simulink model "nn_fuel_control_3_15"  (R2021a)
settings: Solver=ode15s  StartTime=0.0  StopTime=T  MaxStep=.01  RelTol=1e-3
undefined symbols (not defined in the file): AF_sensor_tol, fault_time, fuel_inj_tol, kappa_tol, MAF_sensor_tol, pump_tol, tau_ww_tol
libraries: neural x50
(part 2 of 2)

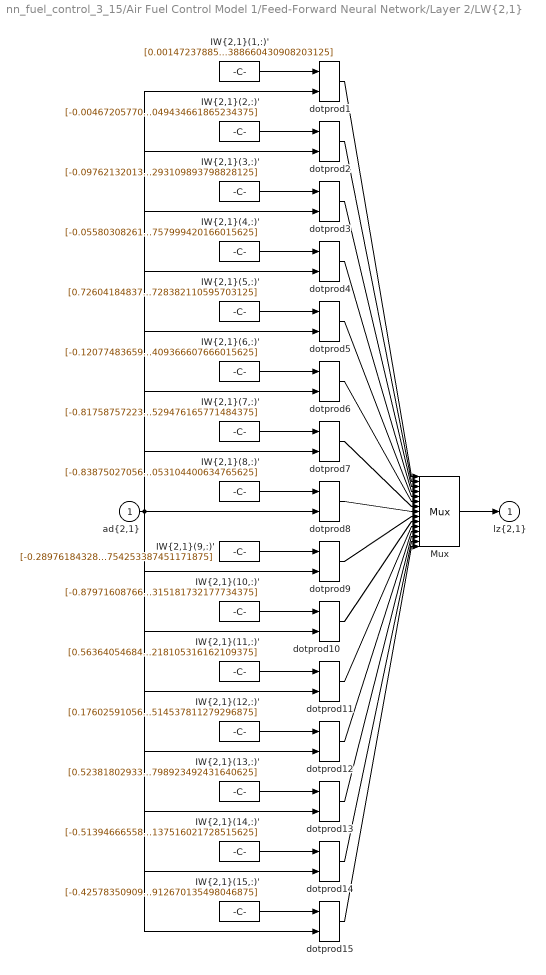
== system nn_fuel_control_3_15/Air Fuel Control Model 1/Feed-Forward Neural Network/Layer 2/LW{2,1} ==
  "ad{2,1}" : Inport  PortDimensions=15
      mask Display: e = 0.06;c1 = [120 230 180]/255;c2 = ([120 230 180]+0)/(256+128);c3 = ([120 230 180]+128)/(256+128);patch([0 1 1 0],[0 0 1 1],c1);patch([0 1 1 1-e 1-e 0+e],[0 0 1 1-e 0+e 0+e],c2);patch([0 0 1 1-e 0+e 0+e],[0 1 1 1-e 1-e 0+e],c3);plot([0 1 1 0 0],[0 0 1 1 0]);
  "IW{2,1}(1,:)'" : Constant  Value=[0.0014723788564683371049568449961952865123748779296875;-0.4105035744953438037185833309195004403591156005859375;0.92504607137404970540472959328326396644115447998046875;-0.13140968467763602944842205033637583255767822265625;0.88617470350879212759309666580520570278167724609375;0.10943690712673904974483463092838064767420291900634765625;0.8357847560107405371354616363532841205596923828125;-0.1424217355145691865647705753872287459671497344970703125;-0.9683741182261533797515085097984410822391510009765625;0.2078972828309095521870375478101777844130992889404296875;-0.141657891245238809485584852154715918004512786865234375;0.2854467052004372451534663923666812479496002197265625;-0.47802444452566505983526212730794213712215423583984375;0.007742822605644341001085440012730032321996986865997314453125;0.7026691591665628067175930482335388660430908203125]
      mask Display: e = 0.06;c1 = [120 150 230]/255;c2 = ([120 150 230]+0)/383;c3 = ([120 150 230]+128)/383;patch([0 1 1 0],[0 0 1 1],c1);patch([0 1 1 1-e 1-e 0+e],[0 0 1 1-e 0+e 0+e],c2);patch([0 0 1 1-e 0+e 0+e],[0 1 1 1-e 1-e 0+e],c3);plot([0 1 1 0 0],[0 0 1 1 0]);disp('weights');
  "IW{2,1}(10,:)'" : Constant  Value=[-0.8797160876685172770095277883228845894336700439453125;0.789339370544755780656487331725656986236572265625;-0.7233137151600008696306076672044582664966583251953125;0.6015191081513704407512932448298670351505279541015625;-0.11263426835994684582775704484447487629950046539306640625;0.8415776576411524434462307908688671886920928955078125;-0.2980449987010034273993142051040194928646087646484375;-0.171843305813586422203798065311275422573089599609375;0.117265923905212565703237714842543937265872955322265625;0.30307170949009909488580660763545893132686614990234375;-0.293941626387824062049958229181356728076934814453125;-0.03082063515976596335121939773671329021453857421875;-0.9050983525641178584209001201088540256023406982421875;-0.99163442468549334307681419886648654937744140625;0.521943270434400030666211023344658315181732177734375]
      mask Display: e = 0.06;c1 = [120 150 230]/255;c2 = ([120 150 230]+0)/383;c3 = ([120 150 230]+128)/383;patch([0 1 1 0],[0 0 1 1],c1);patch([0 1 1 1-e 1-e 0+e],[0 0 1 1-e 0+e 0+e],c2);patch([0 0 1 1-e 0+e 0+e],[0 1 1 1-e 1-e 0+e],c3);plot([0 1 1 0 0],[0 0 1 1 0]);disp('weights');
  "IW{2,1}(11,:)'" : Constant  Value=[0.5636405468410743413443242388893850147724151611328125;-0.6000555782086010037090773039381019771099090576171875;-0.9083589997321432907284588509355671703815460205078125;-0.039439145748280335368463056511245667934417724609375;-0.360599567968600986933580543336574919521808624267578125;-0.9013962864403468611129710552631877362728118896484375;0.818131379099671374177660254645161330699920654296875;0.2148021088713241433243439360012416727840900421142578125;-0.6090730591420296935467604271252639591693878173828125;-0.490614841968887549494837685415404848754405975341796875;0.87058254048700034477548115319223143160343170166015625;0.9743140261337905894123423422570340335369110107421875;-0.231388861045130678206760421744547784328460693359375;-0.81143184376103416610703789046965539455413818359375;0.7149273616405726894384997649467550218105316162109375]
      mask Display: e = 0.06;c1 = [120 150 230]/255;c2 = ([120 150 230]+0)/383;c3 = ([120 150 230]+128)/383;patch([0 1 1 0],[0 0 1 1],c1);patch([0 1 1 1-e 1-e 0+e],[0 0 1 1-e 0+e 0+e],c2);patch([0 0 1 1-e 0+e 0+e],[0 1 1 1-e 1-e 0+e],c3);plot([0 1 1 0 0],[0 0 1 1 0]);disp('weights');
  "IW{2,1}(12,:)'" : Constant  Value=[0.176025910561064424797450556070543825626373291015625;0.8938959851841807857653066093917004764080047607421875;0.23024565712716604792831276427023112773895263671875;0.5912002453814280134025693769217468798160552978515625;-0.13767899499483693404044970520772039890289306640625;0.39561104597748197875262121669948101043701171875;-0.551936271474654294166839463287033140659332275390625;-0.3033516443932107176095769318635575473308563232421875;-0.7286060567887997496683283316087909042835235595703125;-0.7412289835134810989103471001726575195789337158203125;0.40006283904586847910422875429503619670867919921875;-0.4572149619781218365943686876562424004077911376953125;-0.92336675575178883690341535839252173900604248046875;0.4141772355500019653362642202409915626049041748046875;-0.697359994923690162949014847981743514537811279296875]
      mask Display: e = 0.06;c1 = [120 150 230]/255;c2 = ([120 150 230]+0)/383;c3 = ([120 150 230]+128)/383;patch([0 1 1 0],[0 0 1 1],c1);patch([0 1 1 1-e 1-e 0+e],[0 0 1 1-e 0+e 0+e],c2);patch([0 0 1 1-e 0+e 0+e],[0 1 1 1-e 1-e 0+e],c3);plot([0 1 1 0 0],[0 0 1 1 0]);disp('weights');
  "IW{2,1}(13,:)'" : Constant  Value=[0.5238180293357050931746243804809637367725372314453125;0.4144582229988842403400894909282214939594268798828125;-0.71210330551954204025832950719632208347320556640625;-0.2764686429265024170121023416868411004543304443359375;0.84370835682129097232717640508781187236309051513671875;-0.58371761794929810651666457488317973911762237548828125;-0.647040471028641928086244661244563758373260498046875;-0.0257292770502409000321630827556873555295169353485107421875;-0.109912687998933000788071012721047736704349517822265625;0.41116241447809154241355145131819881498813629150390625;-0.55283670379326566024502653817762620747089385986328125;0.7529229726831230262718008816591463983058929443359375;0.15049080269142611765431638559675775468349456787109375;-0.231897338961606302998319506514235399663448333740234375;-0.070382914756523806687482647248543798923492431640625]
      mask Display: e = 0.06;c1 = [120 150 230]/255;c2 = ([120 150 230]+0)/383;c3 = ([120 150 230]+128)/383;patch([0 1 1 0],[0 0 1 1],c1);patch([0 1 1 1-e 1-e 0+e],[0 0 1 1-e 0+e 0+e],c2);patch([0 0 1 1-e 0+e 0+e],[0 1 1 1-e 1-e 0+e],c3);plot([0 1 1 0 0],[0 0 1 1 0]);disp('weights');
  "IW{2,1}(14,:)'" : Constant  Value=[-0.5139466655833884178861126201809383928775787353515625;-0.6994970916207192690450256122858263552188873291015625;0.02461016033035413885787789922687807120382785797119140625;-0.2071609556260745055311645046458579599857330322265625;0.62690154518222629409507362652220763266086578369140625;-0.68570881908632952406179583704215474426746368408203125;0.6935255351681650637374332291074097156524658203125;0.2274889095578533637631579722437891177833080291748046875;-0.1208011883769616046091499583781114779412746429443359375;0.61407664799677508238318068833905272185802459716796875;-0.860561180678970583102227465133182704448699951171875;-0.901805715626496695591640673228539526462554931640625;-0.756946189561250815103221611934714019298553466796875;0.2377717869806747208460961928722099401056766510009765625;-0.9584754628916682950290351072908379137516021728515625]
      mask Display: e = 0.06;c1 = [120 150 230]/255;c2 = ([120 150 230]+0)/383;c3 = ([120 150 230]+128)/383;patch([0 1 1 0],[0 0 1 1],c1);patch([0 1 1 1-e 1-e 0+e],[0 0 1 1-e 0+e 0+e],c2);patch([0 0 1 1-e 0+e 0+e],[0 1 1 1-e 1-e 0+e],c3);plot([0 1 1 0 0],[0 0 1 1 0]);disp('weights');
  "IW{2,1}(15,:)'" : Constant  Value=[-0.4257835090962220903065826860256493091583251953125;0.7545482545397168561152057009167037904262542724609375;0.693650957176581872687393115484155714511871337890625;-0.6058271909569750146573596794041804969310760498046875;-0.92243298192882450248220038702129386365413665771484375;0.463413219568864220843096290991525165736675262451171875;0.338649245461934089718170071137137711048126220703125;0.484763807823216097414587011371622793376445770263671875;0.39292867758759653096234387703589163720607757568359375;0.805180629601002895157080274657346308231353759765625;0.2171358898594655528757613183188368566334247589111328125;-0.84680999387249666909838197170756757259368896484375;-0.3689431272830090424719173824996687471866607666015625;-0.62736288244411664294375441386364400386810302734375;-0.1978189326577559636888281602296046912670135498046875]
      mask Display: e = 0.06;c1 = [120 150 230]/255;c2 = ([120 150 230]+0)/383;c3 = ([120 150 230]+128)/383;patch([0 1 1 0],[0 0 1 1],c1);patch([0 1 1 1-e 1-e 0+e],[0 0 1 1-e 0+e 0+e],c2);patch([0 0 1 1-e 0+e 0+e],[0 1 1 1-e 1-e 0+e],c3);plot([0 1 1 0 0],[0 0 1 1 0]);disp('weights');
  "IW{2,1}(2,:)'" : Constant  Value=[-0.004672057704449006365621244185604155063629150390625;0.9755623302918092765168012192589230835437774658203125;-0.2802782291596883634809955765376798808574676513671875;0.530568769281649199598405175493098795413970947265625;-0.3711149592822611253950526588596403598785400390625;-0.6701597425193110968422161022317595779895782470703125;0.48671231916720270049836472026072442531585693359375;-0.7434126313786528772453721103374846279621124267578125;-0.153098699941905724841717528761364519596099853515625;0.85133638949894674397000926546752452850341796875;0.9338773130103581454619643409387208521366119384765625;0.8820582695436858244875111267901957035064697265625;-0.9020048816383496870230374042876064777374267578125;-0.32054209486867168976687025860883295536041259765625;-0.5428806493898130636210908050998114049434661865234375]
      mask Display: e = 0.06;c1 = [120 150 230]/255;c2 = ([120 150 230]+0)/383;c3 = ([120 150 230]+128)/383;patch([0 1 1 0],[0 0 1 1],c1);patch([0 1 1 1-e 1-e 0+e],[0 0 1 1-e 0+e 0+e],c2);patch([0 0 1 1-e 0+e 0+e],[0 1 1 1-e 1-e 0+e],c3);plot([0 1 1 0 0],[0 0 1 1 0]);disp('weights');
  "IW{2,1}(3,:)'" : Constant  Value=[-0.097621320133909339489264311851002275943756103515625;0.2612783169119214932152317487634718418121337890625;-0.055215070832447997462022470926967798732221126556396484375;0.8160125298612683764076791703701019287109375;0.65646477091284527460857134428806602954864501953125;-0.19085913401025933477939133808831684291362762451171875;0.3087414420961487326877659143065102398395538330078125;0.9224876971971227579416563457925803959369659423828125;-0.266571874563814203984435380334616638720035552978515625;0.6702336279486582615305678700678981840610504150390625;0.197265872962691324321582442280487157404422760009765625;-0.57729764225107604858067134045995771884918212890625;-0.791492072672669966237890548654831945896148681640625;0.81667830492291937360960218938998878002166748046875;-0.8911950061504072539975140898604877293109893798828125]
      mask Display: e = 0.06;c1 = [120 150 230]/255;c2 = ([120 150 230]+0)/383;c3 = ([120 150 230]+128)/383;patch([0 1 1 0],[0 0 1 1],c1);patch([0 1 1 1-e 1-e 0+e],[0 0 1 1-e 0+e 0+e],c2);patch([0 0 1 1-e 0+e 0+e],[0 1 1 1-e 1-e 0+e],c3);plot([0 1 1 0 0],[0 0 1 1 0]);disp('weights');
  "IW{2,1}(4,:)'" : Constant  Value=[-0.0558030826137325686175927330623380839824676513671875;0.4347023464860020336431034593260847032070159912109375;0.275440674566879317719525488428189419209957122802734375;-0.25350814443316949109430424869060516357421875;0.381186478547256124560504986220621503889560699462890625;-0.53969236281862009718679473735392093658447265625;0.3138820723565487469386425800621509552001953125;0.314206063773635080327295554525335319340229034423828125;-0.91256989931503273982826840438065119087696075439453125;-0.75671300750665537737660315542598254978656768798828125;-0.1656127582319334712313008139972225762903690338134765625;0.4185309459959771771764280856586992740631103515625;-0.76890276522204448195196846427279524505138397216796875;0.661584923547618330985642387531697750091552734375;-0.3590957813671791232223995393724180757999420166015625]
      mask Display: e = 0.06;c1 = [120 150 230]/255;c2 = ([120 150 230]+0)/383;c3 = ([120 150 230]+128)/383;patch([0 1 1 0],[0 0 1 1],c1);patch([0 1 1 1-e 1-e 0+e],[0 0 1 1-e 0+e 0+e],c2);patch([0 0 1 1-e 0+e 0+e],[0 1 1 1-e 1-e 0+e],c3);plot([0 1 1 0 0],[0 0 1 1 0]);disp('weights');
  "IW{2,1}(5,:)'" : Constant  Value=[0.7260418483791071242450243516941554844379425048828125;-0.2323204701209327094346690500969998538494110107421875;0.58094310317328190507168983458541333675384521484375;-0.10149087657121658168080102768726646900177001953125;0.017385472622406965281793844724234077148139476776123046875;-0.2465918696556105016437498989034793339669704437255859375;-0.065147713611995783367092371918261051177978515625;0.82285250893895656165710761342779733240604400634765625;-0.5632819611943988835633945200243033468723297119140625;-0.79200473782083558038635828779661096632480621337890625;-0.58294595380808889029111696800100617110729217529296875;0.8069688237247607531799076241441071033477783203125;-0.5731754303914218251492229683208279311656951904296875;0.74394758108042580158070222751121036708354949951171875;0.757136590987837809763050245237536728382110595703125]
      mask Display: e = 0.06;c1 = [120 150 230]/255;c2 = ([120 150 230]+0)/383;c3 = ([120 150 230]+128)/383;patch([0 1 1 0],[0 0 1 1],c1);patch([0 1 1 1-e 1-e 0+e],[0 0 1 1-e 0+e 0+e],c2);patch([0 0 1 1-e 0+e 0+e],[0 1 1 1-e 1-e 0+e],c3);plot([0 1 1 0 0],[0 0 1 1 0]);disp('weights');
  "IW{2,1}(6,:)'" : Constant  Value=[-0.1207748365903345000305080247926525771617889404296875;-0.4566001292990182758302353249746374785900115966796875;0.7674321577875711231087052510702051222324371337890625;0.532782020818384882687723802519030869007110595703125;-0.5503302152362241628225092426873743534088134765625;-0.870981104051296473045340462704189121723175048828125;-0.3023547547324063611284827857161872088909149169921875;0.2357299472378218130330651547410525381565093994140625;0.71943294959485815098787497845478355884552001953125;0.892178685051398634442421098356135189533233642578125;-0.264484462101378436926779613713733851909637451171875;0.6035938989327063186607347233803011476993560791015625;0.0123594330541221264496698495349846780300140380859375;-0.00799278345603138262731590657494962215423583984375;-0.71855220021363752636034405441023409366607666015625]
      mask Display: e = 0.06;c1 = [120 150 230]/255;c2 = ([120 150 230]+0)/383;c3 = ([120 150 230]+128)/383;patch([0 1 1 0],[0 0 1 1],c1);patch([0 1 1 1-e 1-e 0+e],[0 0 1 1-e 0+e 0+e],c2);patch([0 0 1 1-e 0+e 0+e],[0 1 1 1-e 1-e 0+e],c3);plot([0 1 1 0 0],[0 0 1 1 0]);disp('weights');
  "IW{2,1}(7,:)'" : Constant  Value=[-0.8175875722366179321198842444573529064655303955078125;-0.905813293112641471083179567358456552028656005859375;-0.3844932577919755178896821234957315027713775634765625;0.2056336354930061727230850010528229176998138427734375;-0.76141972218104125857962571899406611919403076171875;-0.9439776643957298318809989723376929759979248046875;0.6997489290599505640244615278788842260837554931640625;0.8655339347746793254856356725213117897510528564453125;0.4664203946738567641006056874175556004047393798828125;0.0626214973472627445261196044157259166240692138671875;0.4649690508771568975276977653265930712223052978515625;-0.38200351988705794070710908272303640842437744140625;-0.666044497810676983107214255142025649547576904296875;0.9083497414519896562268286288599483668804168701171875;-0.0908783258153691431147080947994254529476165771484375]
      mask Display: e = 0.06;c1 = [120 150 230]/255;c2 = ([120 150 230]+0)/383;c3 = ([120 150 230]+128)/383;patch([0 1 1 0],[0 0 1 1],c1);patch([0 1 1 1-e 1-e 0+e],[0 0 1 1-e 0+e 0+e],c2);patch([0 0 1 1-e 0+e 0+e],[0 1 1 1-e 1-e 0+e],c3);plot([0 1 1 0 0],[0 0 1 1 0]);disp('weights');
  "IW{2,1}(8,:)'" : Constant  Value=[-0.8387502705666316504817814347916282713413238525390625;-0.9869927371518103509373531778692267835140228271484375;-0.049215002141873132046612226986326277256011962890625;-0.6725714957969464169451612178818322718143463134765625;-0.41634711954292225044582664850167930126190185546875;-0.0546792633337906952561979778693057596683502197265625;0.067250214964079901847071596421301364898681640625;0.953326667743251920938973853481002151966094970703125;0.6229317567947276756967767141759395599365234375;-0.1667857881477574633066751630394719541072845458984375;-0.302637442651685351080459440709091722965240478515625;-0.318939224670099275016355022671632468700408935546875;-0.370195463658054446653977720416150987148284912109375;0.7529451504205637579758558786124922335147857666015625;-0.6522425522147179410836770330206491053104400634765625]
      mask Display: e = 0.06;c1 = [120 150 230]/255;c2 = ([120 150 230]+0)/383;c3 = ([120 150 230]+128)/383;patch([0 1 1 0],[0 0 1 1],c1);patch([0 1 1 1-e 1-e 0+e],[0 0 1 1-e 0+e 0+e],c2);patch([0 0 1 1-e 0+e 0+e],[0 1 1 1-e 1-e 0+e],c3);plot([0 1 1 0 0],[0 0 1 1 0]);disp('weights');
  "IW{2,1}(9,:)'" : Constant  Value=[-0.289761843282438036339954123832285404205322265625;0.729056578900638907470010963152162730693817138671875;-0.9706045169635231228966176786343567073345184326171875;0.048643020949121318352581511135213077068328857421875;-0.801736747087760104335529831587336957454681396484375;0.146439016247541520243657942046411335468292236328125;0.01347836954570791334617751999758183956146240234375;-0.9838465929090622896779905204311944544315338134765625;0.4562838024232658273859897235524840652942657470703125;0.6070860692817594550518833784735761582851409912109375;0.07218184308062092213731375522911548614501953125;-0.1888803349396008801619473160826601088047027587890625;0.137583839945973007701240931055508553981781005859375;0.8143066908040064166840465986751951277256011962890625;-0.7898209168288345960462493167142383754253387451171875]
      mask Display: e = 0.06;c1 = [120 150 230]/255;c2 = ([120 150 230]+0)/383;c3 = ([120 150 230]+128)/383;patch([0 1 1 0],[0 0 1 1],c1);patch([0 1 1 1-e 1-e 0+e],[0 0 1 1-e 0+e 0+e],c2);patch([0 0 1 1-e 0+e 0+e],[0 1 1 1-e 1-e 0+e],c3);plot([0 1 1 0 0],[0 0 1 1 0]);disp('weights');
  Mux : Mux  Inputs=15
      mask Display: e = 0.06;c1 = [120 150 230]/255;c2 = ([120 150 230]+0)/383;c3 = ([120 150 230]+128)/383;patch([0 1 1 0],[0 0 1 1],c1);patch([0 1 1 1-e 1-e 0+e],[0 0 1 1-e 0+e 0+e],c2);patch([0 0 1 1-e 0+e 0+e],[0 1 1 1-e 1-e 0+e],c3);plot([0 1 1 0 0],[0 0 1 1 0]);disp('Mux');
  dotprod{1..15} (15 alike) : neural/Weight Functions/dotprod
  "lz{2,1}" : Outport
      mask Display: e = 0.06;c1 = [120 230 180]/255;c2 = ([120 230 180]+0)/(256+128);c3 = ([120 230 180]+128)/(256+128);patch([0 1 1 0],[0 0 1 1],c1);patch([0 1 1 1-e 1-e 0+e],[0 0 1 1-e 0+e 0+e],c2);patch([0 0 1 1-e 0+e 0+e],[0 1 1 1-e 1-e 0+e],c3);plot([0 1 1 0 0],[0 0 1 1 0]);
  wires:
  "IW{2,1}(1,:)'"/1 -> dotprod1/1
  "ad{2,1}"/1 -> dotprod1/2, dotprod2/2, dotprod3/2, dotprod4/2, dotprod5/2, dotprod6/2, dotprod7/2, dotprod8/2, dotprod9/2, dotprod10/2, dotprod11/2, dotprod12/2, dotprod13/2, dotprod14/2, dotprod15/2
  dotprod1/1 -> Mux/1
  "IW{2,1}(2,:)'"/1 -> dotprod2/1
  dotprod2/1 -> Mux/2
  "IW{2,1}(3,:)'"/1 -> dotprod3/1
  dotprod3/1 -> Mux/3
  "IW{2,1}(4,:)'"/1 -> dotprod4/1
  dotprod4/1 -> Mux/4
  "IW{2,1}(5,:)'"/1 -> dotprod5/1
  dotprod5/1 -> Mux/5
  "IW{2,1}(6,:)'"/1 -> dotprod6/1
  dotprod6/1 -> Mux/6
  "IW{2,1}(7,:)'"/1 -> dotprod7/1
  dotprod7/1 -> Mux/7
  "IW{2,1}(8,:)'"/1 -> dotprod8/1
  dotprod8/1 -> Mux/8
  "IW{2,1}(9,:)'"/1 -> dotprod9/1
  dotprod9/1 -> Mux/9
  "IW{2,1}(10,:)'"/1 -> dotprod10/1
  dotprod10/1 -> Mux/10
  "IW{2,1}(11,:)'"/1 -> dotprod11/1
  dotprod11/1 -> Mux/11
  "IW{2,1}(12,:)'"/1 -> dotprod12/1
  dotprod12/1 -> Mux/12
  "IW{2,1}(13,:)'"/1 -> dotprod13/1
  dotprod13/1 -> Mux/13
  "IW{2,1}(14,:)'"/1 -> dotprod14/1
  dotprod14/1 -> Mux/14
  "IW{2,1}(15,:)'"/1 -> dotprod15/1
  dotprod15/1 -> Mux/15
  Mux/1 -> "lz{2,1}"/1

== system nn_fuel_control_3_15/Air Fuel Control Model 1/Feed-Forward Neural Network/Layer 3/Delays 1 ==
  "p{3}" : Inport  PortDimensions=15
      mask Display: e = 0.06;c1 = [120 230 180]/255;c2 = ([120 230 180]+0)/(256+128);c3 = ([120 230 180]+128)/(256+128);patch([0 1 1 0],[0 0 1 1],c1);patch([0 1 1 1-e 1-e 0+e],[0 0 1 1-e 0+e 0+e],c2);patch([0 0 1 1-e 0+e 0+e],[0 1 1 1-e 1-e 0+e],c3);plot([0 1 1 0 0],[0 0 1 1 0]);
  mux : Mux  Inputs=1
      mask Display: e = 0.06;c1 = [120 150 230]/255;c2 = ([120 150 230]+0)/383;c3 = ([120 150 230]+128)/383;patch([0 1 1 0],[0 0 1 1],c1);patch([0 1 1 1-e 1-e 0+e],[0 0 1 1-e 0+e 0+e],c2);patch([0 0 1 1-e 0+e 0+e],[0 1 1 1-e 1-e 0+e],c3);plot([0 1 1 0 0],[0 0 1 1 0]);disp('Mux')
  "pd{3,2}" : Outport
      mask Display: e = 0.06;c1 = [120 230 180]/255;c2 = ([120 230 180]+0)/(256+128);c3 = ([120 230 180]+128)/(256+128);patch([0 1 1 0],[0 0 1 1],c1);patch([0 1 1 1-e 1-e 0+e],[0 0 1 1-e 0+e 0+e],c2);patch([0 0 1 1-e 0+e 0+e],[0 1 1 1-e 1-e 0+e],c3);plot([0 1 1 0 0],[0 0 1 1 0]);
  wires:
  "p{3}"/1 -> mux/1
  mux/1 -> "pd{3,2}"/1

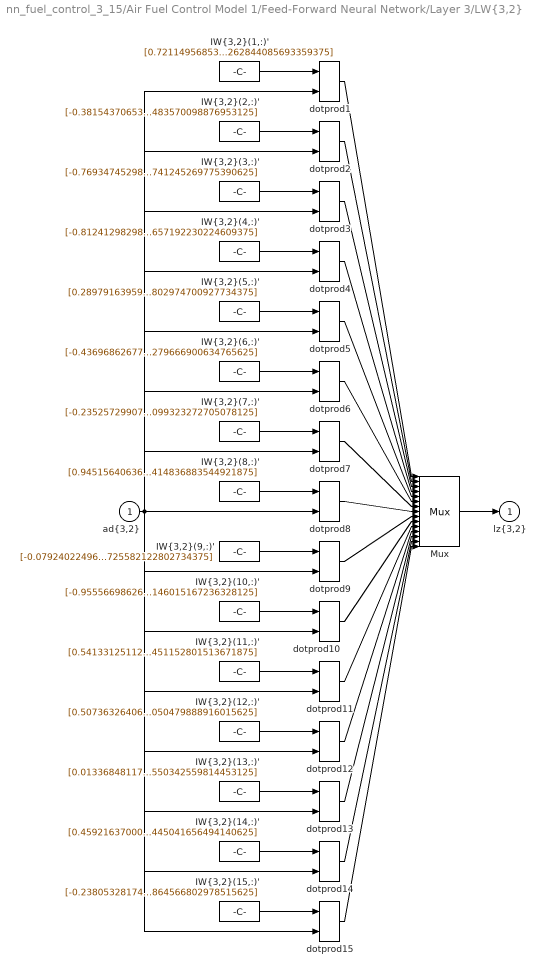
== system nn_fuel_control_3_15/Air Fuel Control Model 1/Feed-Forward Neural Network/Layer 3/LW{3,2} ==
  "ad{3,2}" : Inport  PortDimensions=15
      mask Display: e = 0.06;c1 = [120 230 180]/255;c2 = ([120 230 180]+0)/(256+128);c3 = ([120 230 180]+128)/(256+128);patch([0 1 1 0],[0 0 1 1],c1);patch([0 1 1 1-e 1-e 0+e],[0 0 1 1-e 0+e 0+e],c2);patch([0 0 1 1-e 0+e 0+e],[0 1 1 1-e 1-e 0+e],c3);plot([0 1 1 0 0],[0 0 1 1 0]);
  "IW{3,2}(1,:)'" : Constant  Value=[0.7211495685398465749216256881481967866420745849609375;-0.1560525184820991118073152392753399908542633056640625;-0.7353140609977757424786659612436778843402862548828125;0.89383587442760958907683743746019899845123291015625;0.7517978237884952452674269807175733149051666259765625;-0.8645074614204755203417107622954063117504119873046875;-0.5271368049894198382077092901454307138919830322265625;-0.82425541716965877725442624068818986415863037109375;-0.6388254815435698841241674017510376870632171630859375;0.3222741257529555536365251100505702197551727294921875;-0.2743698476465035174243212168221361935138702392578125;0.3018688161945790593421179437427781522274017333984375;-0.6124294514765964425606625809450633823871612548828125;0.053171224200661004744006277178414165973663330078125;-0.924368960870477707203463069163262844085693359375]
      mask Display: e = 0.06;c1 = [120 150 230]/255;c2 = ([120 150 230]+0)/383;c3 = ([120 150 230]+128)/383;patch([0 1 1 0],[0 0 1 1],c1);patch([0 1 1 1-e 1-e 0+e],[0 0 1 1-e 0+e 0+e],c2);patch([0 0 1 1-e 0+e 0+e],[0 1 1 1-e 1-e 0+e],c3);plot([0 1 1 0 0],[0 0 1 1 0]);disp('weights');
  "IW{3,2}(10,:)'" : Constant  Value=[-0.9555669862685267634816455029067583382129669189453125;0.394863125416177407345230676583014428615570068359375;-0.8520224955936603894457448404864408075809478759765625;-0.225951935749418186816228626412339508533477783203125;0.631217772021331224863160969107411801815032958984375;-0.8237425820303092560692448387271724641323089599609375;-0.0564082446703031425982999280677177011966705322265625;-0.91240172135808705888848635368049144744873046875;-0.744800544642146622464906613458879292011260986328125;-0.976070843861260417639869046979583799839019775390625;-0.5455127760820925875151488071423955261707305908203125;0.0153911770564241212611023001954890787601470947265625;0.53770406203590237481648728135041892528533935546875;-0.4194345530953160761100662057287991046905517578125;0.5690741806895858179160541112651117146015167236328125]
      mask Display: e = 0.06;c1 = [120 150 230]/255;c2 = ([120 150 230]+0)/383;c3 = ([120 150 230]+128)/383;patch([0 1 1 0],[0 0 1 1],c1);patch([0 1 1 1-e 1-e 0+e],[0 0 1 1-e 0+e 0+e],c2);patch([0 0 1 1-e 0+e 0+e],[0 1 1 1-e 1-e 0+e],c3);plot([0 1 1 0 0],[0 0 1 1 0]);disp('weights');
  "IW{3,2}(11,:)'" : Constant  Value=[0.5413312511294143813955770383472554385662078857421875;0.70632467122050446306502635707147419452667236328125;-0.3807065228012571633797733738902024924755096435546875;0.3517480021825145630742781577282585203647613525390625;-0.4236771228098719088706047841696999967098236083984375;-0.6516701658588111012448962355847470462322235107421875;0.1169621799832769593052717027603648602962493896484375;-0.284334984661937628658279209048487246036529541015625;0.3701534462136442105162359439418651163578033447265625;0.6621363257911732080884803508524782955646514892578125;-0.2163558644540206632456147417542524635791778564453125;-0.57005143438306493663958463002927601337432861328125;-0.924562163857749030881905127898789942264556884765625;-0.7829828161563188171356841849046759307384490966796875;0.824633687084030508884779919753782451152801513671875]
      mask Display: e = 0.06;c1 = [120 150 230]/255;c2 = ([120 150 230]+0)/383;c3 = ([120 150 230]+128)/383;patch([0 1 1 0],[0 0 1 1],c1);patch([0 1 1 1-e 1-e 0+e],[0 0 1 1-e 0+e 0+e],c2);patch([0 0 1 1-e 0+e 0+e],[0 1 1 1-e 1-e 0+e],c3);plot([0 1 1 0 0],[0 0 1 1 0]);disp('weights');
  "IW{3,2}(12,:)'" : Constant  Value=[0.507363264064779162509921661694534122943878173828125;-0.292115174483057682408571054111234843730926513671875;0.513324654934169899433982209302484989166259765625;-0.5837418080754954718969429450226016342639923095703125;-0.953780108028102091566324816085398197174072265625;0.2187928995518306773959693600772880017757415771484375;-0.06677646643976942186782252974808216094970703125;-0.93885633069739871103820405551232397556304931640625;0.2998349758037708312485847272910177707672119140625;-0.8896170821201720979587435067514888942241668701171875;0.1267267837731991253491514726192690432071685791015625;0.631327861968670855929985918919555842876434326171875;-0.4416459209828340615189290474518202245235443115234375;-0.41356298509924105388790849247016012668609619140625;0.20287619416835500629758826107718050479888916015625]
      mask Display: e = 0.06;c1 = [120 150 230]/255;c2 = ([120 150 230]+0)/383;c3 = ([120 150 230]+128)/383;patch([0 1 1 0],[0 0 1 1],c1);patch([0 1 1 1-e 1-e 0+e],[0 0 1 1-e 0+e 0+e],c2);patch([0 0 1 1-e 0+e 0+e],[0 1 1 1-e 1-e 0+e],c3);plot([0 1 1 0 0],[0 0 1 1 0]);disp('weights');
  "IW{3,2}(13,:)'" : Constant  Value=[0.013368481177302153628527747741827624849975109100341796875;-0.323601064657340398156293304054997861385345458984375;-0.3727497600216291839814175546052865684032440185546875;0.0707149214661739466958323419021326117217540740966796875;0.58106740396620282229633858150918968021869659423828125;-0.812636642629665839621111445012502372264862060546875;-0.6019297525288085370931412398931570351123809814453125;-0.218586335284584265536977909505367279052734375;-0.467426775396174942756033487967215478420257568359375;0.53489317279096282309325260939658619463443756103515625;0.29980818134041709033255074245971627533435821533203125;-0.5202617895023646799046446176362223923206329345703125;0.837938935714360955131496666581369936466217041015625;0.9207784689598226268714142861426807940006256103515625;-0.80602869221515949238465736925718374550342559814453125]
      mask Display: e = 0.06;c1 = [120 150 230]/255;c2 = ([120 150 230]+0)/383;c3 = ([120 150 230]+128)/383;patch([0 1 1 0],[0 0 1 1],c1);patch([0 1 1 1-e 1-e 0+e],[0 0 1 1-e 0+e 0+e],c2);patch([0 0 1 1-e 0+e 0+e],[0 1 1 1-e 1-e 0+e],c3);plot([0 1 1 0 0],[0 0 1 1 0]);disp('weights');
  "IW{3,2}(14,:)'" : Constant  Value=[0.4592163700034797013671550303115509450435638427734375;-0.780987176718388464990994179970584809780120849609375;-0.75068584783817815520023941644467413425445556640625;0.927478570310972916246328168199397623538970947265625;0.43642317428064902884443654329515993595123291015625;-0.5740108704863466915213621177827008068561553955078125;-0.0110900874857573494836060490342788398265838623046875;-0.21534183571391185552101887878961861133575439453125;-0.6300518694994250434859850429347716271877288818359375;-0.9587528450169238158906637181644327938556671142578125;0.2751982028582229400370806615683250129222869873046875;-0.2137846091583452956541577805182896554470062255859375;-0.88022886393703547724953750730492174625396728515625;-0.1326925671652576799175449195900000631809234619140625;-0.452560522025765354925397332408465445041656494140625]
      mask Display: e = 0.06;c1 = [120 150 230]/255;c2 = ([120 150 230]+0)/383;c3 = ([120 150 230]+128)/383;patch([0 1 1 0],[0 0 1 1],c1);patch([0 1 1 1-e 1-e 0+e],[0 0 1 1-e 0+e 0+e],c2);patch([0 0 1 1-e 0+e 0+e],[0 1 1 1-e 1-e 0+e],c3);plot([0 1 1 0 0],[0 0 1 1 0]);disp('weights');
  "IW{3,2}(15,:)'" : Constant  Value=[-0.2380532817442225501647357077672495506703853607177734375;-0.8861899422655812319504775587120093405246734619140625;0.285818823451112036249099901397130452096462249755859375;-0.0117642649452553184341585534866680973209440708160400390625;-0.444057625906285113881466486418503336608409881591796875;0.3696725590584934995064259055652655661106109619140625;-0.81657758258134993667454182286746799945831298828125;-0.3157676611838329261416902227210812270641326904296875;0.154217722729583339713599343667738139629364013671875;-0.86227035331503032455913171361316926777362823486328125;0.9268425612284938441831627642386592924594879150390625;-0.4029303353404973808693512182799167931079864501953125;0.556506149069358801995122121297754347324371337890625;-0.7100155684251425736164264890248887240886688232421875;0.436614619073472154386905685896635986864566802978515625]
      mask Display: e = 0.06;c1 = [120 150 230]/255;c2 = ([120 150 230]+0)/383;c3 = ([120 150 230]+128)/383;patch([0 1 1 0],[0 0 1 1],c1);patch([0 1 1 1-e 1-e 0+e],[0 0 1 1-e 0+e 0+e],c2);patch([0 0 1 1-e 0+e 0+e],[0 1 1 1-e 1-e 0+e],c3);plot([0 1 1 0 0],[0 0 1 1 0]);disp('weights');
  "IW{3,2}(2,:)'" : Constant  Value=[-0.38154370653407976288207237303140573203563690185546875;-0.0973816884273450700248986322549171745777130126953125;-0.4236406370685441569179374710074625909328460693359375;-0.6517247772070948741429674555547535419464111328125;-0.96336917810215771940107742921099998056888580322265625;0.8362371241085539974591256395797245204448699951171875;0.1788792245088794974350321353995241224765777587890625;0.700588858847600359780471990234218537807464599609375;0.48004187258607000643451101495884358882904052734375;0.54175556645345801509705552234663628041744232177734375;0.83201274429840810231695513721206225454807281494140625;0.8613371062784793696920360162039287388324737548828125;0.9970233159218204743723390492959879338741302490234375;0.360262901958021963810807619665865786373615264892578125;-0.06049054534730842480616530565384891815483570098876953125]
      mask Display: e = 0.06;c1 = [120 150 230]/255;c2 = ([120 150 230]+0)/383;c3 = ([120 150 230]+128)/383;patch([0 1 1 0],[0 0 1 1],c1);patch([0 1 1 1-e 1-e 0+e],[0 0 1 1-e 0+e 0+e],c2);patch([0 0 1 1-e 0+e 0+e],[0 1 1 1-e 1-e 0+e],c3);plot([0 1 1 0 0],[0 0 1 1 0]);disp('weights');
  "IW{3,2}(3,:)'" : Constant  Value=[-0.76934745298175333250156882058945484459400177001953125;0.874520749580145473345282880472950637340545654296875;0.8743310254391978286747644233400933444499969482421875;-0.68583090005516134102236947001074440777301788330078125;-0.82474673260217545855965681766974739730358123779296875;0.5405527278799568957623478127061389386653900146484375;0.149951720395176568700890129548497498035430908203125;-0.5910409368644582439600299039739184081554412841796875;0.6570108155327865073758175640250556170940399169921875;0.7278837510550502098993774779955856502056121826171875;-0.1060752703040962752201181729105883277952671051025390625;-0.9912588626555034476695027478854171931743621826171875;0.720541504544838229406877871952019631862640380859375;-0.62962171500544983349101357816834934055805206298828125;0.0120582844311295823980234587224913411773741245269775390625]
      mask Display: e = 0.06;c1 = [120 150 230]/255;c2 = ([120 150 230]+0)/383;c3 = ([120 150 230]+128)/383;patch([0 1 1 0],[0 0 1 1],c1);patch([0 1 1 1-e 1-e 0+e],[0 0 1 1-e 0+e 0+e],c2);patch([0 0 1 1-e 0+e 0+e],[0 1 1 1-e 1-e 0+e],c3);plot([0 1 1 0 0],[0 0 1 1 0]);disp('weights');
  "IW{3,2}(4,:)'" : Constant  Value=[-0.812412982989143994672076587448827922344207763671875;0.422017339172002348135492866276763379573822021484375;0.59865231375103977740081973024643957614898681640625;-0.360510998509423696845033191493712365627288818359375;-0.30668827075477500532230124008492566645145416259765625;-0.3381728190339945427922430098988115787506103515625;0.5808575976790526507187450988567434251308441162109375;0.2865150581147093422629268388845957815647125244140625;0.8223771538690238802615795066230930387973785400390625;0.462228699617662497356462836251012049615383148193359375;-0.83590224548127978199119070268352515995502471923828125;-0.262731144464245058856022296822629868984222412109375;-0.043771374339012548981830974526019417680799961090087890625;0.4092045521455691670098531176336109638214111328125;0.5456638208272044376911935614771209657192230224609375]
      mask Display: e = 0.06;c1 = [120 150 230]/255;c2 = ([120 150 230]+0)/383;c3 = ([120 150 230]+128)/383;patch([0 1 1 0],[0 0 1 1],c1);patch([0 1 1 1-e 1-e 0+e],[0 0 1 1-e 0+e 0+e],c2);patch([0 0 1 1-e 0+e 0+e],[0 1 1 1-e 1-e 0+e],c3);plot([0 1 1 0 0],[0 0 1 1 0]);disp('weights');
  "IW{3,2}(5,:)'" : Constant  Value=[0.2897916395926467547639049371355213224887847900390625;0.931451804372600111747715345700271427631378173828125;-0.8625221467993482438174623894155956804752349853515625;-0.9522461930130072804701057975762523710727691650390625;-0.3121127987857448271569182907114736735820770263671875;-0.004359894255910656823971294215880334377288818359375;-0.410943526245755474946008689585141837596893310546875;-0.695406824712994531267895581549964845180511474609375;-0.388440910279419515660492834285832941532135009765625;0.9725665588460425947658904988202266395092010498046875;-0.518686296067577767843204128439538180828094482421875;-0.404421122916839070882133455597795546054840087890625;-0.4297445703570830222162157951970584690570831298828125;0.368587032736791275766563558136112987995147705078125;-0.4240103023024541784025132074020802974700927734375]
      mask Display: e = 0.06;c1 = [120 150 230]/255;c2 = ([120 150 230]+0)/383;c3 = ([120 150 230]+128)/383;patch([0 1 1 0],[0 0 1 1],c1);patch([0 1 1 1-e 1-e 0+e],[0 0 1 1-e 0+e 0+e],c2);patch([0 0 1 1-e 0+e 0+e],[0 1 1 1-e 1-e 0+e],c3);plot([0 1 1 0 0],[0 0 1 1 0]);disp('weights');
  "IW{3,2}(6,:)'" : Constant  Value=[-0.43696862677298364818767595352255739271640777587890625;-0.444038545649029448014744048123247921466827392578125;0.97369451538098406029320130983251146972179412841796875;-0.1464578238907616736241834587417542934417724609375;-0.70170966725883887615822231964557431638240814208984375;-0.264639363012559858390204681199975311756134033203125;-0.158324089598124384536959041724912822246551513671875;-0.4072739052543583593291032229899428784847259521484375;0.1615702003464545288835552128148265182971954345703125;0.1066543693493474387334885022937669418752193450927734375;0.1775279498653928034190840890005347318947315216064453125;-0.342572374293284465096576241194270551204681396484375;0.41424309117134072710797454419662244617938995361328125;-0.6536947120514173814598279932397417724132537841796875;0.50078627999508873447354062591330148279666900634765625]
      mask Display: e = 0.06;c1 = [120 150 230]/255;c2 = ([120 150 230]+0)/383;c3 = ([120 150 230]+128)/383;patch([0 1 1 0],[0 0 1 1],c1);patch([0 1 1 1-e 1-e 0+e],[0 0 1 1-e 0+e 0+e],c2);patch([0 0 1 1-e 0+e 0+e],[0 1 1 1-e 1-e 0+e],c3);plot([0 1 1 0 0],[0 0 1 1 0]);disp('weights');
  "IW{3,2}(7,:)'" : Constant  Value=[-0.23525729907094927728650191056658513844013214111328125;-0.2294795014308028680005691057885996997356414794921875;0.39736683074053480435594565278734080493450164794921875;0.169461137909198866768889502054662443697452545166015625;0.052211962547497776931937352173918043263256549835205078125;0.48489382733068442377089013461954891681671142578125;0.3556682279463323492763038302655331790447235107421875;0.0559580177785330423745335792773403227329254150390625;0.7681819055656777806007085018791258335113525390625;0.5446738983438066394882071108440868556499481201171875;0.8359972475625501164842034995672293007373809814453125;-0.545329549954302716940901518682949244976043701171875;0.52068561043953931477545893358183093369007110595703125;0.59231571386508730103770403729868121445178985595703125;-0.76234755002281240354733427011524327099323272705078125]
      mask Display: e = 0.06;c1 = [120 150 230]/255;c2 = ([120 150 230]+0)/383;c3 = ([120 150 230]+128)/383;patch([0 1 1 0],[0 0 1 1],c1);patch([0 1 1 1-e 1-e 0+e],[0 0 1 1-e 0+e 0+e],c2);patch([0 0 1 1-e 0+e 0+e],[0 1 1 1-e 1-e 0+e],c3);plot([0 1 1 0 0],[0 0 1 1 0]);disp('weights');
  "IW{3,2}(8,:)'" : Constant  Value=[0.9451564063655819580844763549976050853729248046875;0.99882633091156147742140092304907739162445068359375;0.7558045769635912680683986764051951467990875244140625;-0.3620003681378662907519583313842304050922393798828125;-0.51223690050787540339882752959965728223323822021484375;0.1258415847760041561542720955912955105304718017578125;-0.91720649183052760378132006735540926456451416015625;-0.4176284006371522306011456748819909989833831787109375;-0.41588607333938920618265910889022052288055419921875;-0.76409864618707967753863385951262898743152618408203125;-0.11298647128678819540059663495412678457796573638916015625;-0.4986278798448406934795684719574637711048126220703125;0.7340595317701661404186097570345737040042877197265625;-0.9338073949096707959682817090651951730251312255859375;-0.12346800698882169633474603642753208987414836883544921875]
      mask Display: e = 0.06;c1 = [120 150 230]/255;c2 = ([120 150 230]+0)/383;c3 = ([120 150 230]+128)/383;patch([0 1 1 0],[0 0 1 1],c1);patch([0 1 1 1-e 1-e 0+e],[0 0 1 1-e 0+e 0+e],c2);patch([0 0 1 1-e 0+e 0+e],[0 1 1 1-e 1-e 0+e],c3);plot([0 1 1 0 0],[0 0 1 1 0]);disp('weights');
  "IW{3,2}(9,:)'" : Constant  Value=[-0.0792402249637979838592372061611968092620372772216796875;0.8653444224772031123649185246904380619525909423828125;-0.40864822739137540708043161430396139621734619140625;-0.2585798102590139979639616285567171871662139892578125;0.8578822926038498497547379884053952991962432861328125;-0.0565659187802383112142479149042628705501556396484375;0.616647321533127179549182983464561402797698974609375;-0.0642592955219927208787566996761597692966461181640625;-0.457374985701640479618390600080601871013641357421875;-0.7297356611383218893962521178764291107654571533203125;-0.2022068540522469481945933011957095004618167877197265625;0.520670769215438422605757295968942344188690185546875;0.332546410485694110548138269223272800445556640625;0.75148268386759842218936000790563412010669708251953125;0.79916333122457583471032194211147725582122802734375]
      mask Display: e = 0.06;c1 = [120 150 230]/255;c2 = ([120 150 230]+0)/383;c3 = ([120 150 230]+128)/383;patch([0 1 1 0],[0 0 1 1],c1);patch([0 1 1 1-e 1-e 0+e],[0 0 1 1-e 0+e 0+e],c2);patch([0 0 1 1-e 0+e 0+e],[0 1 1 1-e 1-e 0+e],c3);plot([0 1 1 0 0],[0 0 1 1 0]);disp('weights');
  Mux : Mux  Inputs=15
      mask Display: e = 0.06;c1 = [120 150 230]/255;c2 = ([120 150 230]+0)/383;c3 = ([120 150 230]+128)/383;patch([0 1 1 0],[0 0 1 1],c1);patch([0 1 1 1-e 1-e 0+e],[0 0 1 1-e 0+e 0+e],c2);patch([0 0 1 1-e 0+e 0+e],[0 1 1 1-e 1-e 0+e],c3);plot([0 1 1 0 0],[0 0 1 1 0]);disp('Mux');
  dotprod{1..15} (15 alike) : neural/Weight Functions/dotprod
  "lz{3,2}" : Outport
      mask Display: e = 0.06;c1 = [120 230 180]/255;c2 = ([120 230 180]+0)/(256+128);c3 = ([120 230 180]+128)/(256+128);patch([0 1 1 0],[0 0 1 1],c1);patch([0 1 1 1-e 1-e 0+e],[0 0 1 1-e 0+e 0+e],c2);patch([0 0 1 1-e 0+e 0+e],[0 1 1 1-e 1-e 0+e],c3);plot([0 1 1 0 0],[0 0 1 1 0]);
  wires:
  "IW{3,2}(1,:)'"/1 -> dotprod1/1
  "ad{3,2}"/1 -> dotprod1/2, dotprod2/2, dotprod3/2, dotprod4/2, dotprod5/2, dotprod6/2, dotprod7/2, dotprod8/2, dotprod9/2, dotprod10/2, dotprod11/2, dotprod12/2, dotprod13/2, dotprod14/2, dotprod15/2
  dotprod1/1 -> Mux/1
  "IW{3,2}(2,:)'"/1 -> dotprod2/1
  dotprod2/1 -> Mux/2
  "IW{3,2}(3,:)'"/1 -> dotprod3/1
  dotprod3/1 -> Mux/3
  "IW{3,2}(4,:)'"/1 -> dotprod4/1
  dotprod4/1 -> Mux/4
  "IW{3,2}(5,:)'"/1 -> dotprod5/1
  dotprod5/1 -> Mux/5
  "IW{3,2}(6,:)'"/1 -> dotprod6/1
  dotprod6/1 -> Mux/6
  "IW{3,2}(7,:)'"/1 -> dotprod7/1
  dotprod7/1 -> Mux/7
  "IW{3,2}(8,:)'"/1 -> dotprod8/1
  dotprod8/1 -> Mux/8
  "IW{3,2}(9,:)'"/1 -> dotprod9/1
  dotprod9/1 -> Mux/9
  "IW{3,2}(10,:)'"/1 -> dotprod10/1
  dotprod10/1 -> Mux/10
  "IW{3,2}(11,:)'"/1 -> dotprod11/1
  dotprod11/1 -> Mux/11
  "IW{3,2}(12,:)'"/1 -> dotprod12/1
  dotprod12/1 -> Mux/12
  "IW{3,2}(13,:)'"/1 -> dotprod13/1
  dotprod13/1 -> Mux/13
  "IW{3,2}(14,:)'"/1 -> dotprod14/1
  dotprod14/1 -> Mux/14
  "IW{3,2}(15,:)'"/1 -> dotprod15/1
  dotprod15/1 -> Mux/15
  Mux/1 -> "lz{3,2}"/1

== system nn_fuel_control_3_15/Air Fuel Control Model 1/Feed-Forward Neural Network/Layer 4/Delays 1 ==
  "p{4}" : Inport  PortDimensions=15
      mask Display: e = 0.06;c1 = [120 230 180]/255;c2 = ([120 230 180]+0)/(256+128);c3 = ([120 230 180]+128)/(256+128);patch([0 1 1 0],[0 0 1 1],c1);patch([0 1 1 1-e 1-e 0+e],[0 0 1 1-e 0+e 0+e],c2);patch([0 0 1 1-e 0+e 0+e],[0 1 1 1-e 1-e 0+e],c3);plot([0 1 1 0 0],[0 0 1 1 0]);
  mux : Mux  Inputs=1
      mask Display: e = 0.06;c1 = [120 150 230]/255;c2 = ([120 150 230]+0)/383;c3 = ([120 150 230]+128)/383;patch([0 1 1 0],[0 0 1 1],c1);patch([0 1 1 1-e 1-e 0+e],[0 0 1 1-e 0+e 0+e],c2);patch([0 0 1 1-e 0+e 0+e],[0 1 1 1-e 1-e 0+e],c3);plot([0 1 1 0 0],[0 0 1 1 0]);disp('Mux')
  "pd{4,3}" : Outport
      mask Display: e = 0.06;c1 = [120 230 180]/255;c2 = ([120 230 180]+0)/(256+128);c3 = ([120 230 180]+128)/(256+128);patch([0 1 1 0],[0 0 1 1],c1);patch([0 1 1 1-e 1-e 0+e],[0 0 1 1-e 0+e 0+e],c2);patch([0 0 1 1-e 0+e 0+e],[0 1 1 1-e 1-e 0+e],c3);plot([0 1 1 0 0],[0 0 1 1 0]);
  wires:
  "p{4}"/1 -> mux/1
  mux/1 -> "pd{4,3}"/1

== system nn_fuel_control_3_15/Air Fuel Control Model 1/Feed-Forward Neural Network/Layer 4/LW{4,3} ==
  "ad{4,3}" : Inport  PortDimensions=15
      mask Display: e = 0.06;c1 = [120 230 180]/255;c2 = ([120 230 180]+0)/(256+128);c3 = ([120 230 180]+128)/(256+128);patch([0 1 1 0],[0 0 1 1],c1);patch([0 1 1 1-e 1-e 0+e],[0 0 1 1-e 0+e 0+e],c2);patch([0 0 1 1-e 0+e 0+e],[0 1 1 1-e 1-e 0+e],c3);plot([0 1 1 0 0],[0 0 1 1 0]);
  "IW{4,3}(1,:)'" : Constant  Value=[0.078502559536130167572309801471419632434844970703125;-0.433818289909333909548649899079464375972747802734375;0.910250791836833883508006692864000797271728515625;-0.374170240884092952793338326955563388764858245849609375;0.1598895125762707092320624724379740655422210693359375;-0.11541565472196145536454281455007730983197689056396484375;0.3439984166464122861128771546646021306514739990234375;-0.48806614017846883246676270573516376316547393798828125;-0.41450170677323450174611707552685402333736419677734375;0.7658138573933757076162009980180300772190093994140625;0.296590572592599688306336247478611767292022705078125;0.764022218577177003595579662942327558994293212890625;0.75288861963462483384290635513025335967540740966796875;0.938498834346770394176928675733506679534912109375;0.733310867269356680964165207115001976490020751953125]
      mask Display: e = 0.06;c1 = [120 150 230]/255;c2 = ([120 150 230]+0)/383;c3 = ([120 150 230]+128)/383;patch([0 1 1 0],[0 0 1 1],c1);patch([0 1 1 1-e 1-e 0+e],[0 0 1 1-e 0+e 0+e],c2);patch([0 0 1 1-e 0+e 0+e],[0 1 1 1-e 1-e 0+e],c3);plot([0 1 1 0 0],[0 0 1 1 0]);disp('weights');
  Mux : Mux  Inputs=1
      mask Display: e = 0.06;c1 = [120 150 230]/255;c2 = ([120 150 230]+0)/383;c3 = ([120 150 230]+128)/383;patch([0 1 1 0],[0 0 1 1],c1);patch([0 1 1 1-e 1-e 0+e],[0 0 1 1-e 0+e 0+e],c2);patch([0 0 1 1-e 0+e 0+e],[0 1 1 1-e 1-e 0+e],c3);plot([0 1 1 0 0],[0 0 1 1 0]);disp('Mux');
  dotprod1 : neural/Weight Functions/dotprod
  "lz{4,3}" : Outport
      mask Display: e = 0.06;c1 = [120 230 180]/255;c2 = ([120 230 180]+0)/(256+128);c3 = ([120 230 180]+128)/(256+128);patch([0 1 1 0],[0 0 1 1],c1);patch([0 1 1 1-e 1-e 0+e],[0 0 1 1-e 0+e 0+e],c2);patch([0 0 1 1-e 0+e 0+e],[0 1 1 1-e 1-e 0+e],c3);plot([0 1 1 0 0],[0 0 1 1 0]);
  wires:
  "IW{4,3}(1,:)'"/1 -> dotprod1/1
  "ad{4,3}"/1 -> dotprod1/2
  dotprod1/1 -> Mux/1
  Mux/1 -> "lz{4,3}"/1
